simulink model "plant"  (R2023a)
settings: configuration reference "config" (kept outside this file)
model workspace (MATLAB code in the model file):
  | cmdLim = Simulink.Parameter;
  | cmdLim.Value = 15;
  | cmdLim.Description = 'Limit for controlling the maximum surface command angle.';
  | cmdLim.Min = 0;
  | cmdLim.Max = 90;
  | cmdLim.DocUnits = 'deg';
  | 
  | dispGain = Simulink.Parameter;
  | dispGain.Value = 0.75;
  | dispGain.Description = 'Gain applied to the displacement error.';
  | dispGain.Min = 0;
  | dispGain.Max = [];
  | dispGain.DocUnits = 'deg/sec/deg';
  | 
  | dispLim = Simulink.Parameter;
  | dispLim.Value = 30;
  | dispLim.Description = 'Limit for controlling the maximum commanded angle.';
  | dispLim.Min = 0;
  | dispLim.Max = 180;
  | dispLim.DocUnits = 'deg';
  | 
  | intGain = Simulink.Parameter;
  | intGain.Value = 0.5;
  | intGain.Description = 'Gain applied to the integral error.';
  | intGain.Min = 0;
  | intGain.Max = [];
  | intGain.DocUnits = 'deg/sec/deg/sec';
  | 
  | intLim = Simulink.Parameter;
  | intLim.Value = 5;
  | intLim.Description = 'Limit for controlling the maximum commanded angle.';
  | intLim.Min = 0;
  | intLim.Max = 90;
  | intLim.DocUnits = 'deg';
  | 
  | rateGain = Simulink.Parameter;
  | rateGain.Value = 2;
  | rateGain.Description = 'Gain applied to the rate error.';
  | rateGain.Min = 0;
  | rateGain.Max = [];
  | rateGain.DocUnits = 'deg/deg/sec';
  | 
  | rateLim = Simulink.Parameter;
  | rateLim.Value = 6;
  | rateLim.Description = 'Limit for controlling the maximum commanded angle.';
  | rateLim.Min = 0;
  | rateLim.Max = 180;
  | rateLim.DocUnits = 'deg/sec';
  | 
  | hdgGain = Simulink.Parameter;
  | hdgGain.Value = 0.015;
settings Model: RequirementInfo={} %GIDa_fe9045fd_0412_4b6e_8206_617cc20e6fde  DataDictionary=model_config.sldd  Creator=Administrator  LastModifiedBy=Administrator
settings ConfigSetRef: SourceName=config

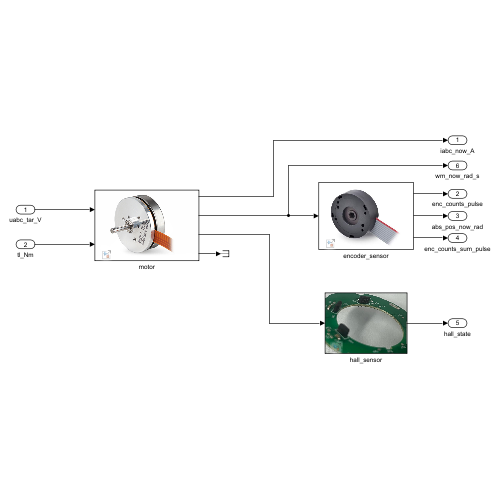
[thumbnail: Simulink's stored preview of the top-level diagram]
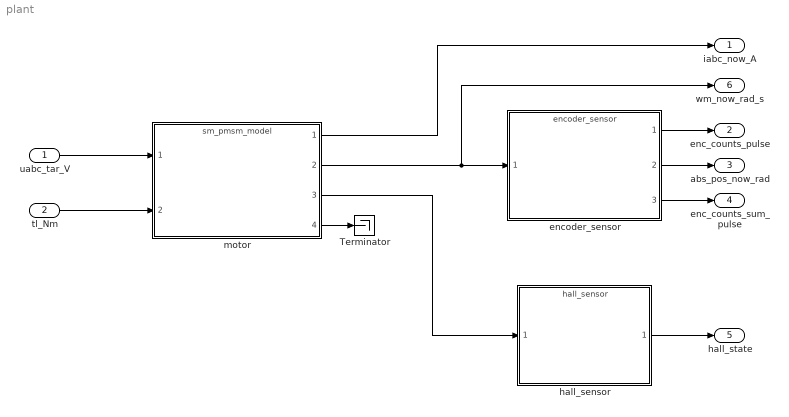
== system plant ==
  uabc_tar_V : Inport
  tl_Nm : Inport  Port=2
  Terminator : Terminator
  encoder_sensor : ModelReference  ModelNameDialog=encoder_sensor.slx  UsingDefaultArgumentValue=0,0,0,0  SimulationMode=Normal  ModelReferenceVersion=1.167
      mask Display: image('$imagefile'); % 使用工具条上的 "编辑图像" 进行更改。
  hall_sensor : ModelReference  ModelNameDialog=hall_sensor.slx  SimulationMode=Normal  ModelReferenceVersion=2.36
      mask Display: image('$imagefile'); % 使用工具条上的 "编辑图像" 进行更改。
  motor : ModelReference  ModelNameDialog=sm_pmsm_model.slx  UsingDefaultArgumentValue=0,0,0,0,0,0,0,0,0,0,0  SimulationMode=Normal  ModelReferenceVersion=1.91
      mask Display: image('D:\class\servo_hub\simulink_project\plant\icon\永磁同步电机.jpg'); % 使用工具条上的 "编辑图像" 进行更改。
  iabc_now_A : Outport
  enc_counts_pulse : Outport  Port=2
  abs_pos_now_rad : Outport  Port=3
  enc_counts_sum_pulse : Outport  Port=4
  hall_state : Outport  Port=5  OutDataTypeStr=uint8
  wm_now_rad_s : Outport  Port=6
  wires:
  motor/3 -> hall_sensor/1
  motor/1 -> iabc_now_A/1
  encoder_sensor/3 -> enc_counts_sum_pulse/1
  motor/2 -> wm_now_rad_s/1, encoder_sensor/1
  encoder_sensor/1 -> enc_counts_pulse/1
  encoder_sensor/2 -> abs_pos_now_rad/1
  hall_sensor/1 -> hall_state/1
  uabc_tar_V/1 -> motor/1
  tl_Nm/1 -> motor/2
  motor/4 -> Terminator/1
